simulink model "gm_mealy_moore_vnl"  (R2016a)
settings: Solver=FixedStepDiscrete  SolverMode=SingleTasking  StartTime=0.0  StopTime=10  RelTol=1e-3
libraries: simulink x5, hdlsllib x4
settings Model: Creator=sande  LastModifiedBy=sande
settings SolverCC: AutoInsertRateTranBlk=on
settings DataIOCC: LimitDataPoints=on  SaveFormat=Array  SaveOutput=off  SaveTime=off
settings OptimizationCC: BlockReduction=off  ConditionallyExecuteInputs=off  DefaultParameterBehavior=Inlined  UseDivisionForNetSlopeComputation=UseDivisionForReciprocalsOfIntegersOnly  UseFloatMulNetSlope=on  InlineInvariantSignals=on  EnhancedBackFolding=on  EfficientFloat2IntCast=on  OptimizeModelRefInitCode=on  LifeSpan=1
settings DebuggingCC: AlgebraicLoopMsg=error  SolverPrmCheckMsg=warning  InheritedTsInSrcMsg=none  SingleTaskRateTransMsg=error  AllowSymbolicDim=off  StrictBusMsg=ErrorOnBusTreatedAsVector  NonBusSignalsTreatedAsBus=error
settings HardwareCC: ProdBitPerPointer=32  ProdLargestAtomicFloat=None  ProdIntDivRoundTo=Undefined  ProdEndianess=Unspecified  ProdWordSize=32  ProdHWDeviceType=ASIC/FPGA->ASIC/FPGA  TargetBitPerPointer=64  TargetLongLongMode=on  TargetIntDivRoundTo=Zero  TargetEndianess=LittleEndian  TargetWordSize=64  TargetHWDeviceType=MATLAB Host  ProdEqTarget=off
settings ModelReferenceCC: PropagateSignalLabelsOutOfModel=off
settings RTWCC: SystemTargetFile=ert.tlc  GenCodeOnly=on  PackageGeneratedCodeAndArtifacts=on  TemplateMakefile=ert_default_tmf  GenerateReport=on  BuildConfiguration=Faster Runs  IncludeHyperlinkInReport=on  LaunchReport=on  TargetLang=C++  GenerateTraceInfo=on  GenerateTraceReport=on  GenerateTraceReportSl=on  GenerateTraceReportSf=on  GenerateTraceReportEml=on  GenerateCodeMetricsReport=on
settings ERTTargetCC: GenerateSampleERTMain=on  CombineSignalStateStructs=on  SuppressErrorStatus=on  MultiInstanceERTCode=on  CodeInterfacePackaging=C++ class  InlinedParameterPlacement=NonHierarchical  RootIOFormat=Structure reference  ERTCustomFileTemplate=example_file_process.tlc  ConvertIfToSwitch=off  SuppressUnreachableDefaultCases=off
settings ConfigComp: CovModelRefEnable=Off  CovSFcnEnable=off

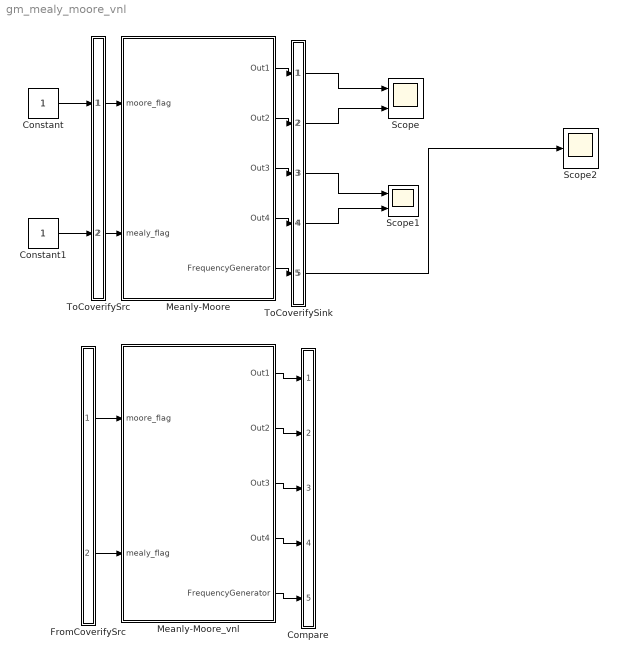
== system gm_mealy_moore_vnl ==
  Compare : Subsystem
      mask Display: disp('')
  Constant : Constant  OutDataTypeStr=boolean  SampleTime=1
  Constant1 : Constant  OutDataTypeStr=boolean  SampleTime=1
  FromCoverifySrc : Subsystem
      mask Display: disp('')
  Meanly-Moore : Subsystem
  Meanly-Moore_vnl : Subsystem
  Scope : Scope  NumInputPorts=2
  Scope1 : Scope  NumInputPorts=2
  Scope2 : Scope
  ToCoverifySink : Subsystem
      mask Display: disp('')
  ToCoverifySrc : Subsystem
      mask Display: disp('')
  wires:
  ToCoverifySrc/1(out1) -> Meanly-Moore/1(moore_flag)
  ToCoverifySrc/2(out2) -> Meanly-Moore/2(mealy_flag)
  Meanly-Moore/1(Out1) -> ToCoverifySink/1(in1)
  Meanly-Moore/2(Out2) -> ToCoverifySink/2(in2)
  Meanly-Moore/3(Out3) -> ToCoverifySink/3(in3)
  Meanly-Moore/4(Out4) -> ToCoverifySink/4(in4)
  Meanly-Moore/5(FrequencyGenerator) -> ToCoverifySink/5(in5)
  Constant/1 -> ToCoverifySrc/1(in1)
  Constant1/1 -> ToCoverifySrc/2(in2)
  ToCoverifySink/1(out1) -> Scope/1
  ToCoverifySink/2(out2) -> Scope/2
  ToCoverifySink/3(out3) -> Scope1/1
  ToCoverifySink/4(out4) -> Scope1/2
  ToCoverifySink/5(out5) -> Scope2/1
  FromCoverifySrc/1(out1) -> Meanly-Moore_vnl/1(moore_flag)
  FromCoverifySrc/2(out2) -> Meanly-Moore_vnl/2(mealy_flag)
  Meanly-Moore_vnl/1(Out1) -> Compare/1(in1)
  Meanly-Moore_vnl/2(Out2) -> Compare/2(in2)
  Meanly-Moore_vnl/3(Out3) -> Compare/3(in3)
  Meanly-Moore_vnl/4(Out4) -> Compare/4(in4)
  Meanly-Moore_vnl/5(FrequencyGenerator) -> Compare/5(in5)

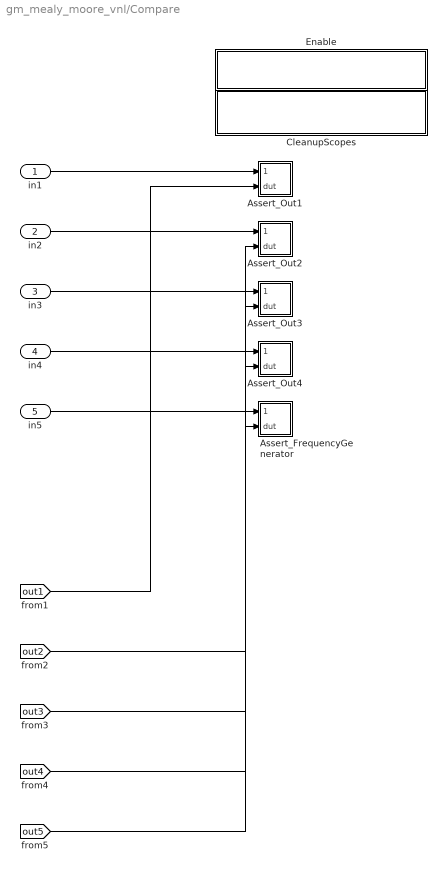
== system gm_mealy_moore_vnl/Compare ==
  in1 : Inport
  in2 : Inport  Port=2
  in3 : Inport  Port=3
  in4 : Inport  Port=4
  in5 : Inport  Port=5
  Assert_FrequencyGenerator : Subsystem
  Assert_Out1 : Subsystem
  Assert_Out2 : Subsystem
  Assert_Out3 : Subsystem
  Assert_Out4 : Subsystem
  CleanupScopes : Subsystem
      settings: OpenFcn=|
      | blkName = gcb; %self block
      | idx = regexp(blkName, '/CleanupScopes$', 'once');
      | blkParent = blkName(1:idx-1);
      | blks=find_system(blkParent, 'blocktype', 'TimeScope');
      | for itr = 1:length(blks)
      | 	 hScopeCfg = get_param(blks{itr},'ScopeConfiguration');
      | 	 hScopeCfg.Visible = ~ hScopeCfg.Visible;
      | end
      | drawnow;
      mask Display: fprintf(message('hdlcoder:cosim:vnl_dblclick').getString());
  Enable : Subsystem
      settings: OpenFcn=|
      | blkName = gcb;
      | idx = regexp(blkName, '/Enable$', 'once');
      | blkParent = blkName(1:idx-1);
      | blks=find_system(blkParent, 'blocktype', 'Assertion');
      | e = get_param(blks{1}, 'Enabled');
      | if strcmp(e, 'on'), f= 'off';, else, f = 'on';, end
      | for ii=1:length(blks), set_param(blks{ii}, 'Enabled', f);, end
      | set_param(gcb, 'MaskDisplay',['fprintf(message(''hdlcoder:cosim:vnl_dblclick_assertions'',','''',upper(e),'''',').getString())']);
      mask Display: fprintf(message('hdlcoder:cosim:vnl_dblclick_assertions','OFF').getString());
  wires:
  in1/1 -> Assert_Out1/1(cosim)
  [out1] -> Assert_Out1/2(dut)
  in2/1 -> Assert_Out2/1(cosim)
  [out2] -> Assert_Out2/2(dut)
  in3/1 -> Assert_Out3/1(cosim)
  [out3] -> Assert_Out3/2(dut)
  in4/1 -> Assert_Out4/1(cosim)
  [out4] -> Assert_Out4/2(dut)
  in5/1 -> Assert_FrequencyGenerator/1(cosim)
  [out5] -> Assert_FrequencyGenerator/2(dut)

== system gm_mealy_moore_vnl/FromCoverifySrc ==
  out1 : Outport
  out2 : Outport  Port=2
  wires:
  [in1] -> out1/1
  [in2] -> out2/1

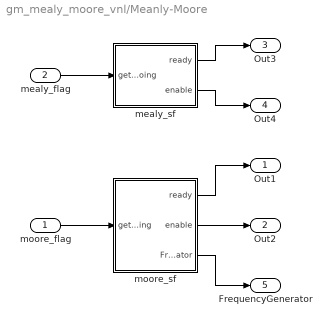
== system gm_mealy_moore_vnl/Meanly-Moore ==
  moore_flag : Inport  OutDataTypeStr=boolean  SampleTime=1
  mealy_flag : Inport  Port=2  OutDataTypeStr=boolean  SampleTime=1
  mealy_sf : Subsystem
  moore_sf : Subsystem
  Out1 : Outport
  Out2 : Outport  Port=2
  Out3 : Outport  Port=3
  Out4 : Outport  Port=4
  FrequencyGenerator : Outport  Port=5
  wires:
  moore_sf/3(FrequencyGenerator) -> FrequencyGenerator/1
  moore_sf/2(enable) -> Out2/1
  moore_sf/1(ready) -> Out1/1
  mealy_sf/2(enable) -> Out4/1
  mealy_sf/1(ready) -> Out3/1
  mealy_flag/1 -> mealy_sf/1(get_going)
  moore_flag/1 -> moore_sf/1(get_going)

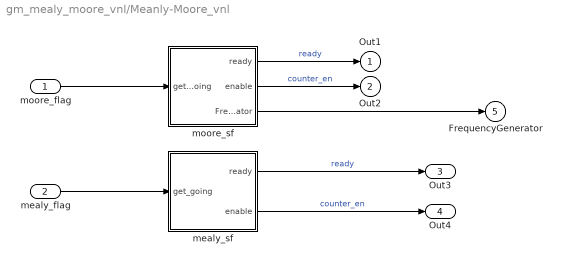
== system gm_mealy_moore_vnl/Meanly-Moore_vnl ==
  moore_flag : Inport
  mealy_flag : Inport  Port=2
  mealy_sf : Subsystem
  moore_sf : Subsystem
  Out1 : Outport
  Out2 : Outport  Port=2
  Out3 : Outport  Port=3
  Out4 : Outport  Port=4
  FrequencyGenerator : Outport  Port=5
  wires:
  moore_sf/3(FrequencyGenerator) -> FrequencyGenerator/1
  mealy_sf/1(ready) -> Out3/1  "ready"
  moore_sf/2(enable) -> Out2/1  "counter_en"
  moore_flag/1 -> moore_sf/1(get_going)
  moore_sf/1(ready) -> Out1/1  "ready"
  mealy_sf/2(enable) -> Out4/1  "counter_en"
  mealy_flag/1 -> mealy_sf/1(get_going)

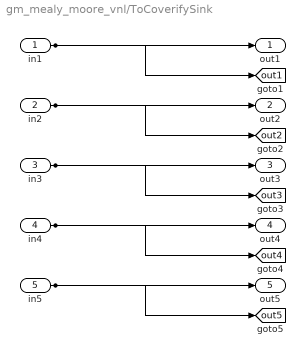
== system gm_mealy_moore_vnl/ToCoverifySink ==
  in1 : Inport
  in2 : Inport  Port=2
  in3 : Inport  Port=3
  in4 : Inport  Port=4
  in5 : Inport  Port=5
  out1 : Outport
  out2 : Outport  Port=2
  out3 : Outport  Port=3
  out4 : Outport  Port=4
  out5 : Outport  Port=5
  tag scope: out1=global, out2=global, out3=global, out4=global, out5=global
  wires:
  in1/1 -> out1/1, [out1]
  in2/1 -> out2/1, [out2]
  in3/1 -> out3/1, [out3]
  in4/1 -> out4/1, [out4]
  in5/1 -> out5/1, [out5]

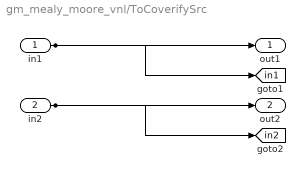
== system gm_mealy_moore_vnl/ToCoverifySrc ==
  in1 : Inport
  in2 : Inport  Port=2
  out1 : Outport
  out2 : Outport  Port=2
  tag scope: in1=global, in2=global
  wires:
  in1/1 -> out1/1, [in1]
  in2/1 -> out2/1, [in2]

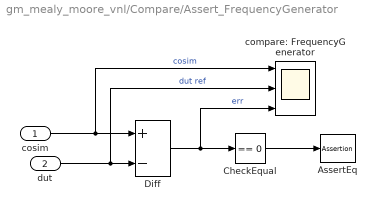
== system gm_mealy_moore_vnl/Compare/Assert_FrequencyGenerator ==
  cosim : Inport
  dut : Inport  Port=2
  AssertEq : Assertion  StopWhenAssertionFail=off
  CheckEqual : simulink/Logic and Bit Operations/Compare To Zero  relop===  OutDataTypeStr=uint8  ZeroCross=off
  Diff : Sum  Inputs=+-
  compare: FrequencyGenerator : Scope  NumInputPorts=3
  wires:
  CheckEqual/1 -> AssertEq/1
  dut/1 -> Diff/2, compare: FrequencyGenerator/2  "dut ref"
  cosim/1 -> compare: FrequencyGenerator/1, Diff/1  "cosim"
  Diff/1 -> CheckEqual/1, compare: FrequencyGenerator/3  "err"

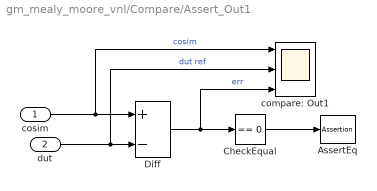
== system gm_mealy_moore_vnl/Compare/Assert_Out1 ==
  cosim : Inport
  dut : Inport  Port=2
  AssertEq : Assertion  StopWhenAssertionFail=off
  CheckEqual : simulink/Logic and Bit Operations/Compare To Zero  relop===  OutDataTypeStr=uint8  ZeroCross=off
  Diff : Sum  Inputs=+-
  compare: Out1 : Scope  NumInputPorts=3
  wires:
  CheckEqual/1 -> AssertEq/1
  dut/1 -> Diff/2, compare: Out1/2  "dut ref"
  cosim/1 -> compare: Out1/1, Diff/1  "cosim"
  Diff/1 -> CheckEqual/1, compare: Out1/3  "err"

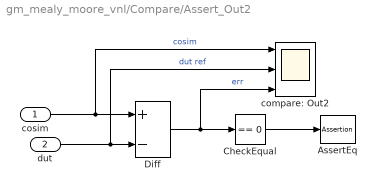
== system gm_mealy_moore_vnl/Compare/Assert_Out2 ==
  cosim : Inport
  dut : Inport  Port=2
  AssertEq : Assertion  StopWhenAssertionFail=off
  CheckEqual : simulink/Logic and Bit Operations/Compare To Zero  relop===  OutDataTypeStr=uint8  ZeroCross=off
  Diff : Sum  Inputs=+-
  compare: Out2 : Scope  NumInputPorts=3
  wires:
  CheckEqual/1 -> AssertEq/1
  dut/1 -> Diff/2, compare: Out2/2  "dut ref"
  cosim/1 -> compare: Out2/1, Diff/1  "cosim"
  Diff/1 -> CheckEqual/1, compare: Out2/3  "err"

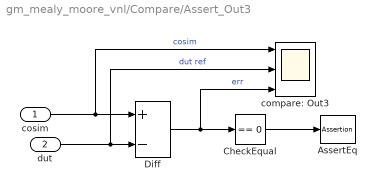
== system gm_mealy_moore_vnl/Compare/Assert_Out3 ==
  cosim : Inport
  dut : Inport  Port=2
  AssertEq : Assertion  StopWhenAssertionFail=off
  CheckEqual : simulink/Logic and Bit Operations/Compare To Zero  relop===  OutDataTypeStr=uint8  ZeroCross=off
  Diff : Sum  Inputs=+-
  compare: Out3 : Scope  NumInputPorts=3
  wires:
  CheckEqual/1 -> AssertEq/1
  dut/1 -> Diff/2, compare: Out3/2  "dut ref"
  cosim/1 -> compare: Out3/1, Diff/1  "cosim"
  Diff/1 -> CheckEqual/1, compare: Out3/3  "err"

== system gm_mealy_moore_vnl/Compare/Assert_Out4 ==
  cosim : Inport
  dut : Inport  Port=2
  AssertEq : Assertion  StopWhenAssertionFail=off
  CheckEqual : simulink/Logic and Bit Operations/Compare To Zero  relop===  OutDataTypeStr=uint8  ZeroCross=off
  Diff : Sum  Inputs=+-
  compare: Out4 : Scope  NumInputPorts=3
  wires:
  CheckEqual/1 -> AssertEq/1
  dut/1 -> Diff/2, compare: Out4/2  "dut ref"
  cosim/1 -> compare: Out4/1, Diff/1  "cosim"
  Diff/1 -> CheckEqual/1, compare: Out4/3  "err"

== system gm_mealy_moore_vnl/Compare/CleanupScopes ==

== system gm_mealy_moore_vnl/Compare/Enable ==

== system gm_mealy_moore_vnl/Meanly-Moore/mealy_sf ==
  get_going : Inport  SampleTime=1
  HDL Counter : hdlsllib/HDL Operations/HDL Counter  CountType=Count limited  CountInit=hex2num('0000000000000000')  CountStep=hex2num('3ff0000000000000')  CountMax=hex2num('4039000000000000')  CountFromType=Initial value  CountFrom=hex2num('0000000000000000')  CountResetPort=off  CountLoadPort=off  CountEnbPort=on  CountDirPort=off  CountDataType=Unsigned  CountWordLen=8  CountFracLen=0  CountSampTime=1
  Simple_Mealy_Chart : Subsystem
  ready : Outport
  enable : Outport  Port=2
  wires:
  Simple_Mealy_Chart/2(count_en) -> enable/1, HDL Counter/1
  Simple_Mealy_Chart/1(ready) -> ready/1
  HDL Counter/1 -> Simple_Mealy_Chart/2(count)
  get_going/1 -> Simple_Mealy_Chart/1(get_going)

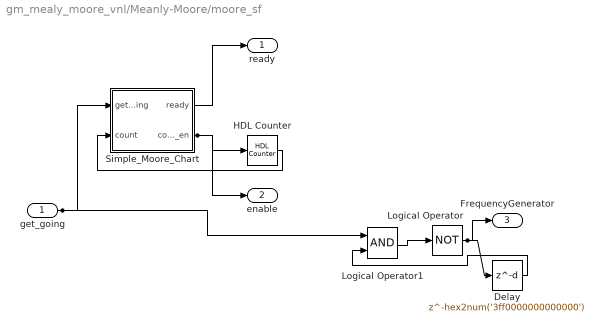
== system gm_mealy_moore_vnl/Meanly-Moore/moore_sf ==
  get_going : Inport  SampleTime=1
  Delay : Delay  DelayLength=hex2num('3ff0000000000000')  InitialCondition=1  InputProcessing=Inherited  SampleTime=1
  HDL Counter : hdlsllib/HDL Operations/HDL Counter  CountType=Count limited  CountInit=hex2num('0000000000000000')  CountStep=hex2num('3ff0000000000000')  CountMax=hex2num('4039000000000000')  CountFromType=Initial value  CountFrom=hex2num('0000000000000000')  CountResetPort=off  CountLoadPort=off  CountEnbPort=on  CountDirPort=off  CountDataType=Unsigned  CountWordLen=8  CountFracLen=0  CountSampTime=1
  Logical Operator : Logic  Operator=NOT  Inputs=1  AllPortsSameDT=off  OutDataTypeStr=boolean  SampleTime=1
  Logical Operator1 : Logic  AllPortsSameDT=off  OutDataTypeStr=boolean  SampleTime=1
  Simple_Moore_Chart : Subsystem
  ready : Outport
  enable : Outport  Port=2
  FrequencyGenerator : Outport  Port=3
  wires:
  Simple_Moore_Chart/2(count_en) -> enable/1, HDL Counter/1
  Simple_Moore_Chart/1(ready) -> ready/1
  Logical Operator1/1 -> Logical Operator/1
  Logical Operator/1 -> FrequencyGenerator/1, Delay/1
  HDL Counter/1 -> Simple_Moore_Chart/2(count)
  Delay/1 -> Logical Operator1/2
  get_going/1 -> Simple_Moore_Chart/1(get_going), Logical Operator1/1

== system gm_mealy_moore_vnl/Meanly-Moore_vnl/mealy_sf ==
  get_going : Inport
  HDL Counter : hdlsllib/HDL Operations/HDL Counter  CountType=Count limited  CountInit=0  CountStep=1  CountMax=25  CountFromType=Initial value  CountFrom=0  CountResetPort=off  CountLoadPort=off  CountEnbPort=on  CountDirPort=off  CountDataType=Unsigned  CountWordLen=8  CountFracLen=0  CountSampTime=1
  Simple_Mealy_Chart : Stateflow chart  TreatAsAtomicUnit=on
  ready : Outport
  enable : Outport  Port=2
  wires:
  HDL Counter/1 -> Simple_Mealy_Chart/2(count)
  Simple_Mealy_Chart/2(count_en) -> enable/1, HDL Counter/1
  Simple_Mealy_Chart/1(ready) -> ready/1  "ready"
  get_going/1 -> Simple_Mealy_Chart/1(get_going)

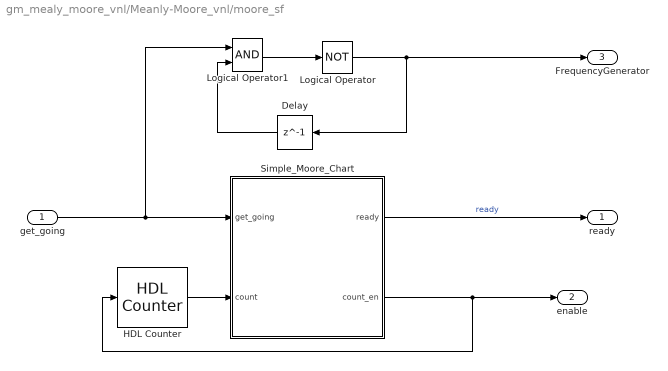
== system gm_mealy_moore_vnl/Meanly-Moore_vnl/moore_sf ==
  get_going : Inport
  Delay : Delay  DelayLength=1  InitialCondition=1
  HDL Counter : hdlsllib/HDL Operations/HDL Counter  CountType=Count limited  CountInit=0  CountStep=1  CountMax=25  CountFromType=Initial value  CountFrom=0  CountResetPort=off  CountLoadPort=off  CountEnbPort=on  CountDirPort=off  CountDataType=Unsigned  CountWordLen=8  CountFracLen=0  CountSampTime=1
  Logical Operator : Logic  Operator=NOT  AllPortsSameDT=off  OutDataTypeStr=boolean
  Logical Operator1 : Logic  AllPortsSameDT=off  OutDataTypeStr=boolean
  Simple_Moore_Chart : Stateflow chart  TreatAsAtomicUnit=on
  ready : Outport
  enable : Outport  Port=2
  FrequencyGenerator : Outport  Port=3
  wires:
  Logical Operator1/1 -> Logical Operator/1
  Delay/1 -> Logical Operator1/2
  Logical Operator/1 -> FrequencyGenerator/1, Delay/1
  get_going/1 -> Simple_Moore_Chart/1(get_going), Logical Operator1/1
  Simple_Moore_Chart/1(ready) -> ready/1  "ready"
  HDL Counter/1 -> Simple_Moore_Chart/2(count)
  Simple_Moore_Chart/2(count_en) -> enable/1, HDL Counter/1

== system gm_mealy_moore_vnl/Meanly-Moore/mealy_sf/Simple_Mealy_Chart ==
  get_going : Inport  SampleTime=1
  count : Inport  Port=2  SampleTime=1
  Simple_Mealy_Chart : Stateflow chart  TreatAsAtomicUnit=on
  ready : Outport
  count_en : Outport  Port=2
  wires:
  Simple_Mealy_Chart/2(count_en) -> count_en/1
  Simple_Mealy_Chart/1(ready) -> ready/1
  count/1 -> Simple_Mealy_Chart/2(count)
  get_going/1 -> Simple_Mealy_Chart/1(get_going)

== system gm_mealy_moore_vnl/Meanly-Moore/moore_sf/Simple_Moore_Chart ==
  get_going : Inport  SampleTime=1
  count : Inport  Port=2  SampleTime=1
  Simple_Moore_Chart : Stateflow chart  TreatAsAtomicUnit=on
  ready : Outport
  count_en : Outport  Port=2
  wires:
  Simple_Moore_Chart/2(count_en) -> count_en/1
  Simple_Moore_Chart/1(ready) -> ready/1
  count/1 -> Simple_Moore_Chart/2(count)
  get_going/1 -> Simple_Moore_Chart/1(get_going)

== stateflow chart gm_mealy_moore_vnl/Meanly-Moore/moore_sf/Simple_Moore_Chart/Simple_Moore_Chart ==
  settings: stateMachineType=MOORE_MACHINE  initializeOutput=1
  state IDLE
    ready = true;
    count_en = false;
  state COUNTING
    ready = false;
    count_en = true;
  (default) -> IDLE
  COUNTING -> IDLE : [(count) == max_count]
  IDLE -> COUNTING : [get_going == true]
  data: get_going input boolean; count input =0; ready output boolean =true; count_en output boolean; max_count constant fixdt(0,5,0) =25

== stateflow chart gm_mealy_moore_vnl/Meanly-Moore/mealy_sf/Simple_Mealy_Chart/Simple_Mealy_Chart ==
  settings: stateMachineType=MEALY_MACHINE  executeAtInitialization=1
  state IDLE
  state COUNTING
  (default) -> IDLE
  COUNTING -> IDLE : [count == max_count]...
      | {ready = true;...
      | count_en = false;}
  IDLE -> COUNTING : [get_going == true]...
      | {ready = false;...
      |  count_en = true;}
  data: get_going input boolean; count input uint8 =0; ready output boolean =true; count_en output boolean; max_count constant uint8 =25

== stateflow chart gm_mealy_moore_vnl/Meanly-Moore_vnl/mealy_sf/Simple_Mealy_Chart ==
  settings: stateMachineType=MEALY_MACHINE  executeAtInitialization=1
  state IDLE
  state COUNTING
  (default) -> IDLE
  COUNTING -> IDLE : [count == max_count]...
      | {ready = true;...
      | count_en = false;}
  IDLE -> COUNTING : [get_going == true]...
      | {ready = false;...
      |  count_en = true;}
  data: get_going input boolean; count input uint8 =0; ready output boolean =true; count_en output boolean; max_count constant uint8 =25

== stateflow chart gm_mealy_moore_vnl/Meanly-Moore_vnl/moore_sf/Simple_Moore_Chart ==
  settings: stateMachineType=MOORE_MACHINE  initializeOutput=1
  state IDLE
    ready = true;
    count_en = false;
  state COUNTING
    ready = false;
    count_en = true;
  (default) -> IDLE
  COUNTING -> IDLE : [(count) == max_count]
  IDLE -> COUNTING : [get_going == true]
  data: get_going input boolean; count input =0; ready output boolean =true; count_en output boolean; max_count constant fixdt(0,5,0) =25
